simulink model "Lab2A"  (R2020a)
settings: Solver=VariableStepAuto  StartTime=0.0  StopTime=9  RelTol=1e-3
libraries: simulink x1
settings Model: Creator=scott  LastModifiedBy=scott

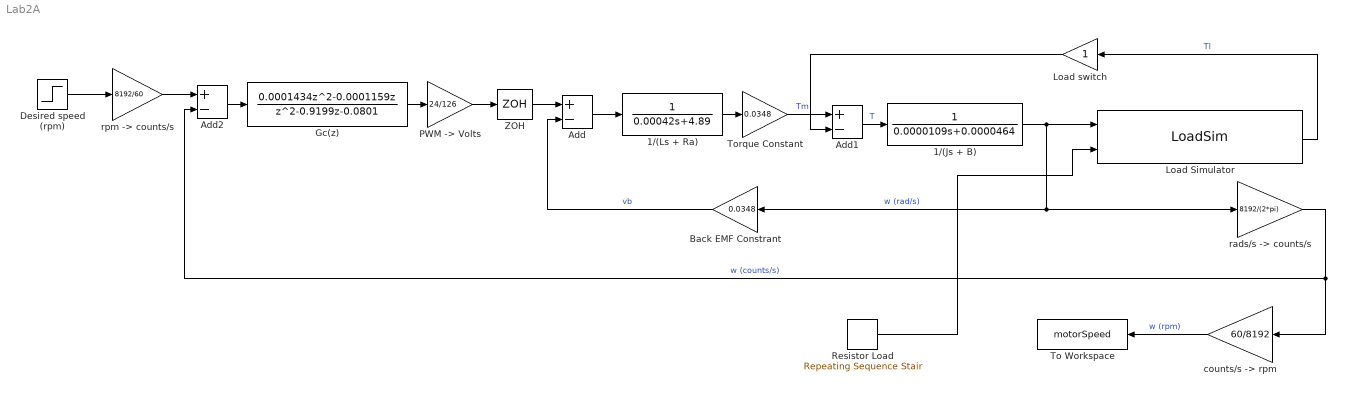
== system Lab2A ==
  1/(Js + B) : TransferFcn  Denominator=[0.0000109 0.0000464]
  1/(Ls + Ra) : TransferFcn  Denominator=[0.00042 4.89]
  Add : Sum  Inputs=+-
  Add1 : Sum  Inputs=+-
  Add2 : Sum  Inputs=+-
  Back EMF Constrant : Gain  Gain=0.0348
  Desired speed (rpm) : Step  Time=0  After=2000  SampleTime=0.008
  Gc(z) : DiscreteTransferFcn  Numerator=[0.0001434 -0.0001159 0]  Denominator=[1 -0.9199 -0.0801]
  "Load Simulator " : S-Function  InitFcn=try, set_param(gcb,'FunctionName','LoadSim'), end  FunctionName=LoadSim  SFunctionModules=LoadSim_wrapper  SFunctionDeploymentMode=off  EnableBusSupport=off  mask(S-Function Builder){}
      mask help: Simulink:masks:SFunctionBuilder_MD
      mask init:
      | val = [[.9  0.75 0.75 1 1 .9 .9 1]',[1 1 0.75 0.75 .9 .9 1 .9]'];try , sys = get_param(gcb,'SfunBuilderFcnName');if isempty(sys), sys = get_param(gcb,'FunctionName'); end,catch, sys = get_param(gcb,'FunctionName'); end
      settings: CopyFcn=set_param(gcbh,'LinkStatus','none')  PreSaveFcn=try, set_param(gcb,'FunctionName','LoadSim'), end  OpenFcn=sfunctionwizard(gcbh)
      mask Display: plot(val(:,1),val(:,2)),disp(sys), port_label('input',1,'omega (rad/s.)'), port_label('input',2,'# of Resistors'), port_label('output',1,'Torque (Nm.)')
  Load switch : Gain
  "PWM -> Volts" : Gain  Gain=24/126
  Resistor Load : simulink/Sources/Repeating Sequence Stair  OutValues=[0 4 14 13 1 6 8].'  tsamp=0.8  OutMin=[]  OutMax=[]  OutDataTypeStr=double  OutputDataTypeScalingMode=double  OutDataType=fixdt(0,8)  ConRadixGroup=Best Precision: Vector-wise  OutScaling=2^-12
  To Workspace : ToWorkspace  VariableName=motorSpeed  SaveFormat=Timeseries  SampleTime=-1
  Torque Constant : Gain  Gain=0.0348
  ZOH : ZeroOrderHold  SampleTime=-1
  "counts/s -> rpm" : Gain  Gain=60/8192
  "rads/s -> counts/s" : Gain  Gain=8192/(2*pi)
  "rpm -> counts/s" : Gain  Gain=8192/60
  wires:
  Add/1 -> 1/(Ls + Ra)/1
  1/(Ls + Ra)/1 -> Torque Constant/1
  Torque Constant/1 -> Add1/1  "Tm"
  Add1/1 -> 1/(Js + B)/1  "T"
  1/(Js + B)/1 -> "Load Simulator "/1, "rads/s -> counts/s"/1, Back EMF Constrant/1  "w (rad/s)"
  "Load Simulator "/1 -> Load switch/1  "Tl"
  Back EMF Constrant/1 -> Add/2  "vb"
  "rads/s -> counts/s"/1 -> "counts/s -> rpm"/1, Add2/2  "w (counts/s)"
  ZOH/1 -> Add/1
  Gc(z)/1 -> "PWM -> Volts"/1
  "PWM -> Volts"/1 -> ZOH/1
  Add2/1 -> Gc(z)/1
  Desired speed (rpm)/1 -> "rpm -> counts/s"/1
  "rpm -> counts/s"/1 -> Add2/1
  Load switch/1 -> Add1/2
  "counts/s -> rpm"/1 -> To Workspace/1  "w (rpm)"
  Resistor Load/1 -> "Load Simulator "/2
